simulink model "D3_LQR_1_QuadrotorModel"  (R2023b)
settings: Solver=VariableStepAuto  StartTime=0.0  StopTime=time_model  RelTol=1e-3
values from neighbouring files (symbols this model uses):
  A_flap = [c_a, c_b, 0 ... (first row only)    [LQR_calculate.m]    (also in LQR_feedback.m; LQR_linearized_test.m; MPC_test.m; MPC_test_1.m)
  A_ind = [c_d, 0, 0 ... (first row only)    [LQR_calculate.m]    (also in LQR_feedback.m; LQR_linearized_test.m; MPC_test.m; MPC_test_1.m)
  C_drag = 0    [LQR_calculate.m]    (also in LQR_feedback.m = C_drag_arr(i); LQR_linearized_test.m = C_drag_arr(i); MPC_test.m = C_drag_arr(i); MPC_test_1.m = C_drag_arr(i))
  demp = 0    [LQR_feedback.m]    (also in LQR_linearized_test.m; MPC_params.m; MPC_test_1.m; initQuadrotorData.m)
  forward_1 = 20    [LQR_feedback.m]    (also in LQR_linearized_test.m; MPC_test_1.m)
  forward_2 = 20    [LQR_feedback.m]    (also in LQR_linearized_test.m; MPC_test_1.m)
  g = 9.81    [LQR_calculate.m]    (also in LQR_feedback.m = 9.8; LQR_linearized_test.m = 9.8; LQR_testing_gpt.m; MPC_params.m = 9.8)
  Ix = m/3*a^2/12+2*0.045*l^2    (= 0.00211347222222)    [LQR_calculate.m]    (also in LQR_feedback.m; LQR_linearized_test.m; LQR_testing_gpt.m = 0.0081; MPC_params.m)
  Iy = m/3*a^2/12+4*0.045*l^2    (= 0.00413847222222)    [LQR_calculate.m]    (also in LQR_feedback.m = 0.00211347222222; LQR_linearized_test.m = 0.00211347222222; LQR_testing_gpt.m = 0.0081; MPC_params.m = 0.00211347222222)
  Iz = m/3*a^2/4+2*0.045*l^2    (= 0.00229041666667)    [LQR_calculate.m]    (also in LQR_feedback.m = 0.00431541666667; LQR_linearized_test.m = 0.00431541666667; LQR_testing_gpt.m = 0.0142; MPC_params.m = 0.00431541666667)
  J = 2.5*10^(-6)    (= 2.5e-06)    [LQR_calculate.m]    (also in LQR_feedback.m; LQR_linearized_test.m; MPC_params.m; MPC_test.m)
  K = Y * inv(P)    [LQR_calculate.m]    (also in LQR_feedback.m = [Kx;Ky;Kz;Kphi;Ktheta;-Kpsi])
  Ke = ke    (= 0.0073)    [LQR_calculate.m]    (also in LQR_feedback.m = 0.00734; LQR_linearized_test.m = 0.00734; MPC_params.m = 0.00734; MPC_test.m)
  kf = ks*r^2*airDensity*Sblade/2    (= 1.57565625e-05)    [LQR_calculate.m]    (also in LQR_feedback.m; LQR_linearized_test.m; MPC_params.m; MPC_test.m)
  Km = kt    (= 0.0073)    [LQR_calculate.m]    (also in LQR_feedback.m = 0.00734; LQR_linearized_test.m = 0.00734; MPC_params.m = 0.00734; MPC_test.m)
  kv = 1300    [LQR_feedback.m]    (also in LQR_linearized_test.m; MPC_test_1.m; initQuadrotorData.m)
  L = La    (= 5e-05)    [LQR_calculate.m]    (also in LQR_feedback.m = 0.0001; LQR_linearized_test.m = 0.0001; MPC_params.m = 0.0001; MPC_test.m)
  l = 0.15    [LQR_calculate.m]    (also in LQR_feedback.m; LQR_linearized_test.m; MPC_params.m; MPC_test.m)
  m = size(B, 2)    [LQR_calculate.m]    (also in LQR_feedback.m = 0.65; LQR_linearized_test.m = 0.65; LQR_testing_gpt.m = 1; MPC_params.m = 0.65)
  Mode = 3    [LQR_feedback.m]    (also in LQR_linearized_test.m; MPC_test_1.m = 1)
  phi0 = 0    [LQR_feedback.m]    (also in LQR_linearized_test.m; MPC_test_1.m)
  psi0 = pi/2    (= 1.57079632679)    [LQR_feedback.m]    (also in LQR_linearized_test.m; MPC_test_1.m = 0)
  R = eye(4)    [LQR_calculate.m]    (also in LQR_feedback.m = 0.058; LQR_linearized_test.m = 0.058; LQR_testing_gpt.m = diag([0.1, 10, 100, 10]); MPC_params.m = 0.058)
  rho = 1.225    [LQR_calculate.m]    (also in LQR_feedback.m; LQR_linearized_test.m; MPC_params.m; MPC_test.m)
  S = l*c*4+a*b    (= 0.0169)    [LQR_calculate.m]    (also in LQR_feedback.m; LQR_linearized_test.m; MPC_params.m; MPC_test.m)
  theta0 = 0    [LQR_feedback.m]    (also in LQR_linearized_test.m; MPC_test_1.m)
  total_time = 60    [LQR_feedback.m]    (also in LQR_linearized_test.m; MPC_test_1.m)
  up_down = 5    [LQR_feedback.m]    (also in LQR_linearized_test.m; MPC_test_1.m)
  x0 = 0    [LQR_feedback.m]    (also in LQR_linearized_test.m; MPC_test_1.m; init_nmpc.m = zeros(nx,1))
  y0 = 0    [LQR_feedback.m]    (also in LQR_linearized_test.m; MPC_test_1.m)
  z0 = 0    [LQR_feedback.m]    (also in LQR_linearized_test.m; MPC_test_1.m)
libraries: vrlib x2, sharedtransform x1
settings Model: Creator=Degra  LastModifiedBy=Degra

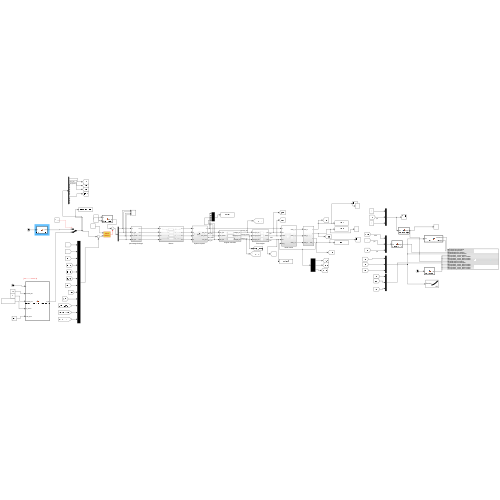
[thumbnail: Simulink's stored preview of the top-level diagram]
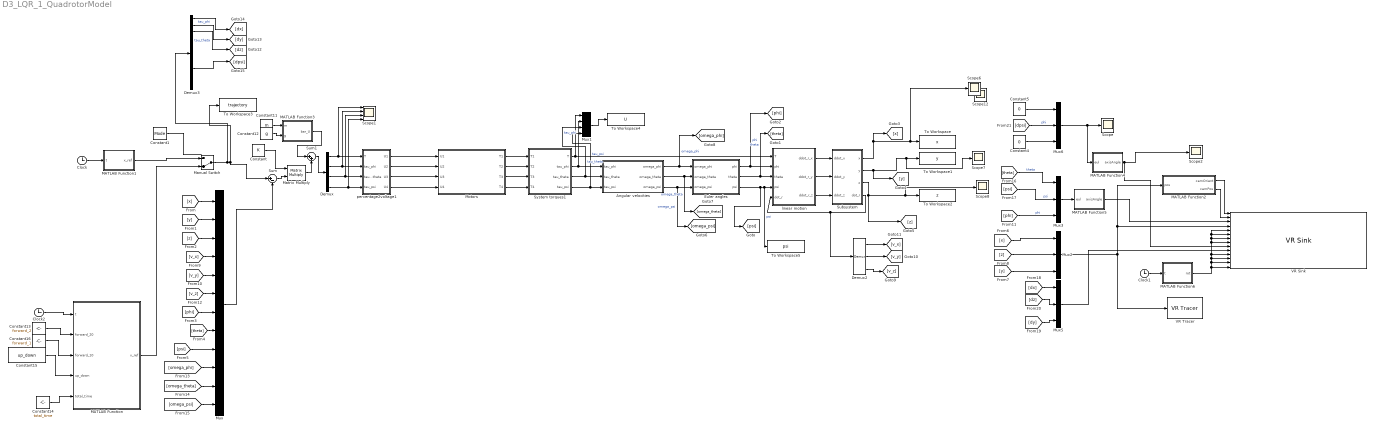
== system D3_LQR_1_QuadrotorModel ==
  Angular velocities : Subsystem
  Clock : Clock
  Clock1 : Clock
  Clock2 : Clock
  Constant : Constant  Value=K
  Constant1 : Constant  Value=Mode
  Constant11 : Constant  Value=m
  Constant12 : Constant  Value=g
  Constant13 : Constant  Value=forward_2
  Constant14 : Constant  Value=total_time
  Constant15 : Constant  Value=up_down
  Constant16 : Constant  Value=forward_1
  Constant4 : Constant  Value=0
  Constant5 : Constant  Value=0
  Demux : Demux
  Demux2 : Demux  Outputs=3
  Demux3 : Demux  Outputs=12
  Euler angles : Subsystem
  MATLAB Function : MATLAB Function  TreatAsAtomicUnit=on
  MATLAB Function1 : MATLAB Function  TreatAsAtomicUnit=on
  MATLAB Function2 : MATLAB Function  TreatAsAtomicUnit=on
  MATLAB Function3 : MATLAB Function  TreatAsAtomicUnit=on
  MATLAB Function4 : MATLAB Function  TreatAsAtomicUnit=on
  MATLAB Function5 : MATLAB Function  TreatAsAtomicUnit=on
  MATLAB Function6 : MATLAB Function  TreatAsAtomicUnit=on
  Manual Switch : ManualSwitch  CurrentSetting=0
  Matrix Multiply : Product  Multiplication=Matrix(*)
  Motors : Subsystem
  Mux : Mux  Inputs=12
  Mux1 : Mux
  Mux{2..3,5..6} (4 alike) : Mux  Inputs=3
  Scope{,2,6..8,12} (6 alike) : Scope
  Scope1 : Scope  NumInputPorts=4
  Subsystem : Subsystem
  Sum : Sum  Inputs=|+-
  Sum1 : Sum  Inputs=|++
  System torques1 : Subsystem
  To Workspace : ToWorkspace  VariableName=x  SaveFormat=Timeseries  SampleTime=-1
  To Workspace1 : ToWorkspace  VariableName=y  SaveFormat=Timeseries  SampleTime=-1
  To Workspace2 : ToWorkspace  VariableName=z  SaveFormat=Timeseries  SampleTime=-1
  To Workspace3 : ToWorkspace  VariableName=trajectory  SaveFormat=Timeseries  SampleTime=-1
  To Workspace4 : ToWorkspace  VariableName=U  SaveFormat=Timeseries  SampleTime=-1
  To Workspace5 : ToWorkspace  VariableName=psi  SaveFormat=Timeseries  SampleTime=-1
  VR Sink : vrlib/VR Sink  InstantiateOnLoad=on  SampleTime=0.1  ViewEnable=on  RemoteChange=off  RemoteView=off  FieldsWritten=FollowCam.orientation.4.1.1.double#FollowCam.position.3.1.1.double#RealQuadrotor.rotation.4.1.1.double#RealQuadrotor.translation.3.1.1.double#Propeller5_center.rotation.4.1.1.double#Propeller5_center_0001.rotation.4.1.1.double#Propeller5_center_0002.rotation.4.1.1.double#Propeller5_center_0003.rotation.4.1.1.double#IdelQuadrotor.rotation.4.1.1.double#IdelQuadrotor.translation.3.1.1.double#Propeller5_center_0004.rotation.4.1.1.double#Propeller5_center_0005.rotation.4.1.1.double#Propeller5_center_0006.rotation.4.1.1.double#Propeller5_center_0007.rotation.4.1.1.double  WorldFileName=quardrotor_space_2.x3d  WorldDescription=Aerodrome in the Desert  AutoView=off  VideoDimensions=[]  AllowVariableSize=off  FigureProperties="{'Position', 'Name', 'Viewpoint', 'CameraBound', 'CameraDirection', 'CameraPosition', 'CameraUpVector', 'ZoomFactor', 'Antialiasing', 'Headlight', 'Lighting', 'NavPanel', 'Sound', 'StatusBar', 'Stereo3D', 'Stereo3DCameraOffset', 'Stereo3DHIT', 'ToolBar', 'Textures', 'Transparency', 'Triad', 'Wireframe', 'NavZones', 'NavMode', 'NavSpeed', 'CaptureFileFormat', 'CaptureFileName', 'Record2DCompressMethod', 'Record2DCompressQuality', 'Record2D', 'Record2DFileName', 'Record2DFPS'; [1.0000000000000000e+00   7.6000000000000000e+01   1.9200000000000000e+03   9.1300000000000000e+02], 'Aerodrome in the Desert', '_untitled_3', 'on', [0.0000000000000000e+00   0.0000000000000000e+00  -1.0000000000000000e+00], [0.0000000000000000e+00   0.0000000000000000e+00   0.0000000000000000e+00], [0.0000000000000000e+00   1.0000000000000000e+00   0.0000000000000000e+00], [1.0000000000000000e+00], 'on', 'on', 'on', 'halfbar', 'on', 'on', 'off', [1.0000000149011612e-01], [0.0000000000000000e+00], 'on', 'on', 'on', 'none', 'off', 'off', 'fly', 'normal', 'tif', '%f_anim_%n.tif', 'auto', [7.5000000000000000e+01], 'on', '%f_anim_%n.avi', 'auto'}"
  VR Tracer : vrlib/VR Tracer  VrmlFile=quardrotor_space_2.x3d  MarkerName=Sphere  UseLines=on  UseTriads=on  MarkerScale=[0.01 0.01 0.01]  MarkerColorSelection=Defined as RGB values  MarkerColor=red  rgbval=[1 0 0]  Ts=0.5  ForceViewerOpen=off  ConnectPlane=off  PlaneCoeff=[0 1 0 0]  ConnectPoint=None  PointCoord=[0 0 0]
  linear motion : Subsystem
  percentage2voltage1 : Subsystem
  wires:
  Angular velocities/1(omega_phi) -> [omega_phi], Euler angles/1(omega_phi)  "omega_phi"
  Angular velocities/2(omega_theta) -> [omega_theta], Euler angles/2(omega_theta)  "omega_theta"
  Angular velocities/3(omega_psi) -> [omega_psi], Euler angles/3(omega_psi)  "omega_psi"
  Euler angles/1(phi) -> [phi], linear motion/2(phi)  "phi"
  Euler angles/2(theta) -> [theta], linear motion/3(theta)  "theta"
  Euler angles/3(psi) -> [psi], To Workspace5/1, linear motion/4(psi)  "psi"
  linear motion/1(ddot_r_x) -> Subsystem/1(ddot_x)
  linear motion/2(ddot_r_y) -> Subsystem/2(ddot_y)
  linear motion/3(ddot_r_z) -> Subsystem/3(ddot_z)
  Subsystem/1(x) -> [x], Scope6/1, To Workspace/1
  Subsystem/2(y) -> [y], Scope7/1, To Workspace1/1
  Subsystem/3(z) -> [z], Scope8/1, To Workspace2/1
  Clock/1 -> MATLAB Function1/1(t)
  [x] -> Mux/1
  [z] -> Mux/3
  [y] -> Mux/2
  Mux/1 -> Sum/2
  [phi] -> Mux/7
  [theta] -> Mux/8
  [psi] -> Mux/9
  [omega_theta] -> Mux/11
  [omega_phi] -> Mux/10
  [omega_psi] -> Mux/12
  [v_z] -> Mux/6
  [v_y] -> Mux/5
  [v_x] -> Mux/4
  Constant/1 -> Matrix Multiply/1
  Sum/1 -> Matrix Multiply/2
  MATLAB Function1/1(x_ref) -> Manual Switch/1
  Constant1/1 -> ?
  ? -> ?
  Demux/1 -> percentage2voltage1/1(T), Scope1/1
  Demux/2 -> percentage2voltage1/2(tau_phi), Scope1/2
  Demux/3 -> percentage2voltage1/3(tau_theta), Scope1/3
  Demux/4 -> percentage2voltage1/4(tau_psi), Scope1/4
  Matrix Multiply/1 -> Sum1/2
  Constant11/1 -> MATLAB Function3/1(m)
  Constant12/1 -> MATLAB Function3/2(g)
  Sum1/1 -> Demux/1
  MATLAB Function3/1(bar_U) -> Sum1/1
  MATLAB Function/1(x_ref) -> Manual Switch/2
  Constant13/1 -> MATLAB Function/2(forward_20)
  Constant16/1 -> MATLAB Function/3(forward_10)
  Constant15/1 -> MATLAB Function/4(up_down)
  Constant14/1 -> MATLAB Function/5(total_time)
  Clock2/1 -> MATLAB Function/1(t)
  Subsystem/4(dot_r) -> Demux2/1, linear motion/5(dot_r)
  Demux2/3 -> [v_z]
  Demux2/2 -> [v_y]
  Demux2/1 -> [v_x]
  System torques1/4(tau_psi) -> Mux1/4, Angular velocities/3(tau_psi)  "tau_psi"
  System torques1/3(tau_theta) -> Mux1/3, Angular velocities/2(tau_theta)  "tau_theta"
  System torques1/2(tau_phi) -> Mux1/2, Angular velocities/1(tau_phi)  "tau_phi"
  System torques1/1(T) -> Mux1/1, linear motion/1(T)
  Motors/1(T1) -> System torques1/1(T1)
  Motors/2(T2) -> System torques1/2(T2)
  Motors/3(T3) -> System torques1/3(T3)
  Motors/4(T4) -> System torques1/4(T4)
  percentage2voltage1/1(U1) -> Motors/1(U1)
  percentage2voltage1/2(U2) -> Motors/2(U2)
  percentage2voltage1/3(U3) -> Motors/3(U3)
  percentage2voltage1/4(U4) -> Motors/4(U4)
  Mux1/1 -> To Workspace4/1
  [x] -> Mux2/1
  [y] -> Mux2/3
  [z] -> Mux2/2
  [phi] -> Mux3/3  "phi"
  Manual Switch/1 -> Demux3/1, Sum/1, To Workspace3/1
  Demux3/3 -> [dz]  "tau_theta"
  Demux3/2 -> [dy]  "tau_phi"
  Demux3/1 -> [dx]
  [dz] -> Mux5/2
  [dy] -> Mux5/3
  [dx] -> Mux5/1
  Mux6/1 -> MATLAB Function4/1(eul), Scope/1
  Mux3/1 -> MATLAB Function5/1(eul)
  Demux3/9 -> [dpsi]
  Constant5/1 -> Mux6/1
  Constant4/1 -> Mux6/3
  MATLAB Function4/1(axisAngle) -> VR Sink/9, Scope2/1
  [psi] -> Mux3/2  "psi"
  [theta] -> Mux3/1  "theta"
  Clock1/1 -> MATLAB Function6/1(t)
  Mux5/1 -> VR Sink/10
  MATLAB Function2/1(camOrient) -> VR Sink/1
  MATLAB Function2/2(camPos) -> VR Sink/2
  MATLAB Function5/1(axisAngle) -> VR Sink/3
  Mux2/1 -> VR Tracer/1, VR Sink/4, MATLAB Function2/1(pos)
  MATLAB Function6/1(rot) -> VR Sink/12, VR Sink/11, VR Sink/8, VR Sink/7, VR Sink/5, VR Sink/6, VR Sink/13, VR Sink/14
  [dpsi] -> Mux6/2  "phi"

== system D3_LQR_1_QuadrotorModel/Angular velocities ==
  tau_phi : Inport
  tau_theta : Inport  Port=2
  tau_psi : Inport  Port=3
  Subsystem1 : Subsystem
  Subsystem2 : Subsystem
  Subsystem3 : Subsystem
  omega_phi : Outport
  omega_theta : Outport  Port=2
  omega_psi : Outport  Port=3
  wires:
  Subsystem2/1(omega_theta) -> omega_theta/1, Subsystem1/2(omega_theta), Subsystem3/3(omega_theta)  "omega_theta"
  tau_theta/1 -> Subsystem2/1(tau_theta)
  Subsystem1/1(omega_phi) -> omega_phi/1, Subsystem3/2(omega_phi), Subsystem2/2(omega_phi)  "omega_phi"
  Subsystem3/1(omega_psi) -> omega_psi/1, Subsystem2/3(omega_psi), Subsystem1/3(omega_psi)  "omega_psi"
  tau_phi/1 -> Subsystem1/1(tau_phi)
  tau_psi/1 -> Subsystem3/1(tau_psi)

== system D3_LQR_1_QuadrotorModel/Euler angles ==
  omega_phi : Inport
  omega_theta : Inport  Port=2
  omega_psi : Inport  Port=3
  Subsystem1 : Subsystem
  Subsystem2 : Subsystem
  Subsystem3 : Subsystem
  phi : Outport
  theta : Outport  Port=2
  psi : Outport  Port=3
  wires:
  Subsystem2/1(theta) -> theta/1, Subsystem1/2(theta), Subsystem3/4(theta)  "theta"
  Subsystem1/1(phi) -> phi/1, Subsystem3/1(phi), Subsystem2/1(phi)  "phi"
  omega_theta/1 -> Subsystem3/2(omega_theta), Subsystem1/3(omega_theta), Subsystem2/2(omega_theta)
  omega_psi/1 -> Subsystem2/3(omega_psi), Subsystem3/3(omega_psi), Subsystem1/4(omega_psi)
  omega_phi/1 -> Subsystem1/1(omega_phi)
  Subsystem3/1(psi) -> psi/1  "psi"

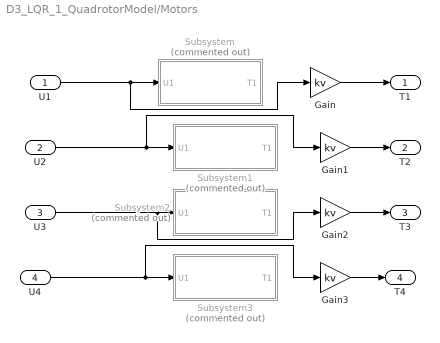
== system D3_LQR_1_QuadrotorModel/Motors ==
  U1 : Inport
  U2 : Inport  Port=2
  U3 : Inport  Port=3
  U4 : Inport  Port=4
  Gain{,1..3} (4 alike) : Gain  Gain=kv
  Subsystem : Subsystem  Commented=on
  Subsystem1 : Subsystem  Commented=on
  Subsystem2 : Subsystem  Commented=on
  Subsystem3 : Subsystem  Commented=on
  T1 : Outport
  T2 : Outport  Port=2
  T3 : Outport  Port=3
  T4 : Outport  Port=4
  wires:
  U4/1 -> Gain3/1, Subsystem3/1(U1)
  U1/1 -> Gain/1, Subsystem/1(U1)
  U3/1 -> Gain2/1, Subsystem2/1(U1)
  U2/1 -> Gain1/1, Subsystem1/1(U1)
  Gain/1 -> T1/1
  Gain1/1 -> T2/1
  Gain2/1 -> T3/1
  Gain3/1 -> T4/1

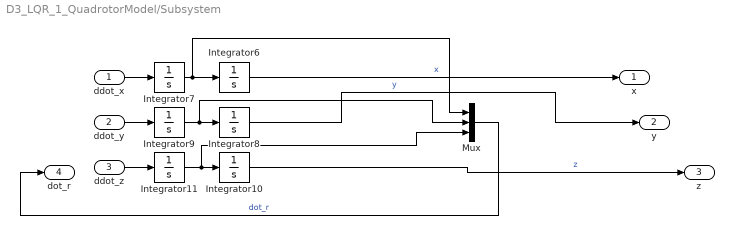
== system D3_LQR_1_QuadrotorModel/Subsystem ==
  ddot_x : Inport
  ddot_y : Inport  Port=2
  ddot_z : Inport  Port=3
  Integrator10 : Integrator  InitialCondition=z0
  Integrator11 : Integrator
  Integrator6 : Integrator  InitialCondition=x0
  Integrator7 : Integrator
  Integrator8 : Integrator  InitialCondition=y0
  Integrator9 : Integrator
  Mux : Mux  Inputs=3
  x : Outport
  y : Outport  Port=2
  z : Outport  Port=3
  dot_r : Outport  Port=4
  wires:
  Integrator9/1 -> Mux/2, Integrator8/1
  Integrator7/1 -> Mux/1, Integrator6/1
  Integrator10/1 -> z/1  "z"
  Integrator11/1 -> Mux/3, Integrator10/1
  Integrator8/1 -> y/1  "y"
  ddot_x/1 -> Integrator7/1
  Mux/1 -> dot_r/1  "dot_r"
  Integrator6/1 -> x/1  "x"
  ddot_y/1 -> Integrator9/1
  ddot_z/1 -> Integrator11/1

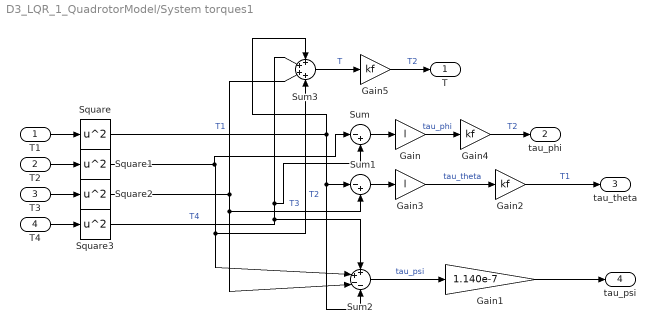
== system D3_LQR_1_QuadrotorModel/System torques1 ==
  T1 : Inport
  T2 : Inport  Port=2
  T3 : Inport  Port=3
  T4 : Inport  Port=4
  Gain : Gain  Gain=l
  Gain1 : Gain  Gain=1.140e-7
  Gain2 : Gain  Gain=kf
  Gain3 : Gain  Gain=l
  Gain4 : Gain  Gain=kf
  Gain5 : Gain  Gain=kf
  Square{,1..3} (4 alike) : Math  Operator=square
  Sum : Sum  Inputs=|-+
  Sum1 : Sum  Inputs=|-+
  Sum2 : Sum  Inputs=++--
  Sum3 : Sum  Inputs=++++
  T : Outport
  tau_phi : Outport  Port=2
  tau_theta : Outport  Port=3
  tau_psi : Outport  Port=4
  wires:
  T3/1 -> Square2/1
  T4/1 -> Square3/1
  Sum2/1 -> Gain1/1  "tau_psi"
  T1/1 -> Square/1
  Sum/1 -> Gain/1
  Sum1/1 -> Gain3/1
  Sum3/1 -> Gain5/1  "T"
  T2/1 -> Square1/1
  Gain3/1 -> Gain2/1  "tau_theta"
  Gain/1 -> Gain4/1  "tau_phi"
  Gain1/1 -> tau_psi/1
  Square/1 -> Sum1/1, Sum2/4, Sum3/1  "T1"
  Square1/1 -> Sum/1, Sum2/2, Sum3/4  "T2"
  Square2/1 -> Sum1/2, Sum2/3, Sum3/3  "T3"
  Square3/1 -> Sum/2, Sum3/2, Sum2/1  "T4"
  Gain4/1 -> tau_phi/1  "T2"
  Gain2/1 -> tau_theta/1  "T1"
  Gain5/1 -> T/1  "T2"

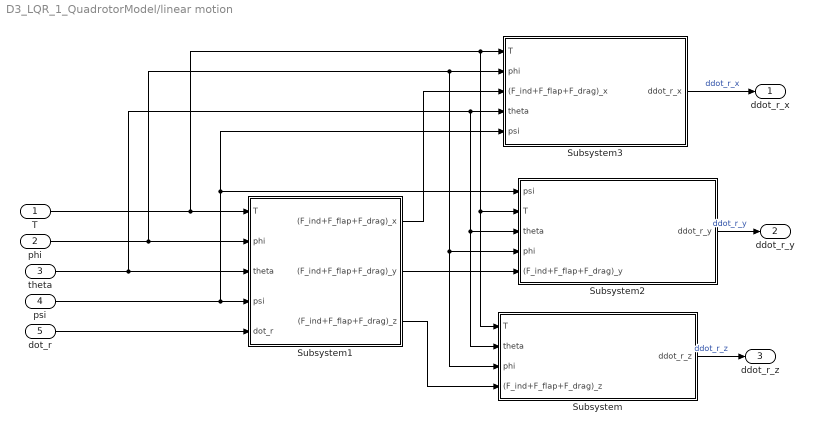
== system D3_LQR_1_QuadrotorModel/linear motion ==
  T : Inport
  phi : Inport  Port=2
  theta : Inport  Port=3
  psi : Inport  Port=4
  dot_r : Inport  Port=5
  Subsystem : Subsystem
  Subsystem1 : Subsystem
  Subsystem2 : Subsystem
  Subsystem3 : Subsystem
  ddot_r_x : Outport
  ddot_r_y : Outport  Port=2
  ddot_r_z : Outport  Port=3
  wires:
  T/1 -> Subsystem/1(T), Subsystem2/2(T), Subsystem3/1(T), Subsystem1/1(T)
  theta/1 -> Subsystem/2(theta), Subsystem2/3(theta), Subsystem3/4(theta), Subsystem1/3(theta)
  phi/1 -> Subsystem/3(phi), Subsystem2/4(phi), Subsystem3/2(phi), Subsystem1/2(phi)
  Subsystem1/3((F_ind+F_flap+F_drag)_z) -> Subsystem/4((F_ind+F_flap+F_drag)_z)
  psi/1 -> Subsystem3/5(psi), Subsystem2/1(psi), Subsystem1/4(psi)
  dot_r/1 -> Subsystem1/5(dot_r)
  Subsystem1/2((F_ind+F_flap+F_drag)_y) -> Subsystem2/5((F_ind+F_flap+F_drag)_y)
  Subsystem1/1((F_ind+F_flap+F_drag)_x) -> Subsystem3/3((F_ind+F_flap+F_drag)_x)
  Subsystem3/1(ddot_r_x) -> ddot_r_x/1  "ddot_r_x"
  Subsystem2/1(ddot_r_y) -> ddot_r_y/1  "ddot_r_y"
  Subsystem/1(ddot_r_z) -> ddot_r_z/1  "ddot_r_z"

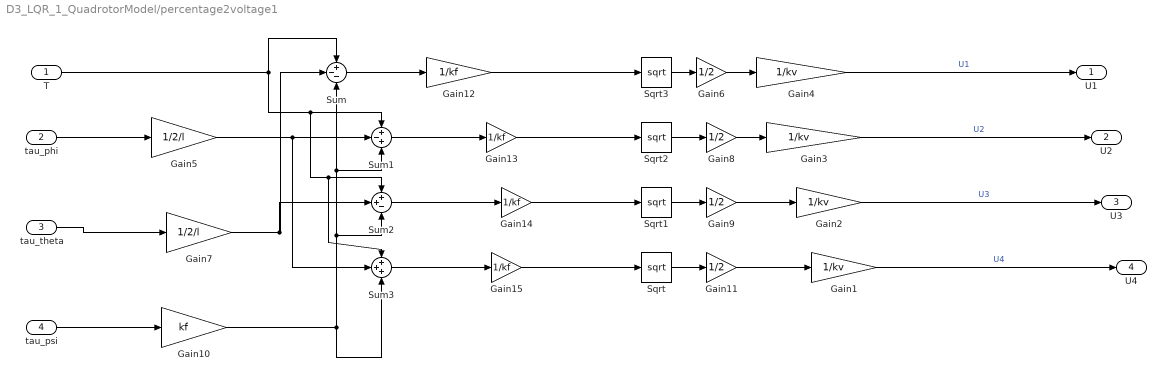
== system D3_LQR_1_QuadrotorModel/percentage2voltage1 ==
  T : Inport
  tau_phi : Inport  Port=2
  tau_theta : Inport  Port=3
  tau_psi : Inport  Port=4
  Gain{1..4} (4 alike) : Gain  Gain=1/kv
  Gain10 : Gain  Gain=kf
  Gain{6,8..9,11} (4 alike) : Gain  Gain=1/2
  Gain{12..15} (4 alike) : Gain  Gain=1/kf
  Gain5 : Gain  Gain=1/2/l
  Gain7 : Gain  Gain=1/2/l
  Sqrt{,1..3} (4 alike) : Sqrt
  Sum : Sum  Inputs=+--
  Sum1 : Sum  Inputs=+-+
  Sum2 : Sum  Inputs=++-
  Sum3 : Sum  Inputs=+++
  U1 : Outport
  U2 : Outport  Port=2
  U3 : Outport  Port=3
  U4 : Outport  Port=4
  wires:
  Gain2/1 -> U3/1  "U3"
  Gain4/1 -> U1/1  "U1"
  Gain3/1 -> U2/1  "U2"
  Gain1/1 -> U4/1  "U4"
  Sum3/1 -> Gain15/1
  Sum2/1 -> Gain14/1
  tau_phi/1 -> Gain5/1
  tau_theta/1 -> Gain7/1
  tau_psi/1 -> Gain10/1
  Gain10/1 -> Sum3/3, Sum1/3, Sum/3, Sum2/3
  Sqrt/1 -> Gain11/1
  Sqrt1/1 -> Gain9/1
  Sqrt2/1 -> Gain8/1
  Sqrt3/1 -> Gain6/1
  Gain6/1 -> Gain4/1
  Gain8/1 -> Gain3/1
  Gain9/1 -> Gain2/1
  Gain11/1 -> Gain1/1
  Sum/1 -> Gain12/1
  Sum1/1 -> Gain13/1
  Gain14/1 -> Sqrt1/1
  Gain15/1 -> Sqrt/1
  Gain5/1 -> Sum3/2, Sum1/2
  Gain7/1 -> Sum2/2, Sum/2
  T/1 -> Sum3/1, Sum2/1, Sum1/1, Sum/1
  Gain12/1 -> Sqrt3/1
  Gain13/1 -> Sqrt2/1

== system D3_LQR_1_QuadrotorModel/Angular velocities/Subsystem1 ==
  tau_phi : Inport
  omega_theta : Inport  Port=2
  omega_psi : Inport  Port=3
  Gain : Gain  Gain=Iy-Iz
  Gain1 : Gain  Gain=1/Ix
  Integrator12 : Integrator
  Product : Product
  Sum : Sum  Inputs=|++
  omega_phi : Outport
  wires:
  Gain/1 -> Sum/2
  omega_theta/1 -> Product/1
  Product/1 -> Gain/1
  Sum/1 -> Gain1/1  "dot_omega_phi"
  tau_phi/1 -> Sum/1
  omega_psi/1 -> Product/2
  Gain1/1 -> Integrator12/1
  Integrator12/1 -> omega_phi/1  "omega_phi"

== system D3_LQR_1_QuadrotorModel/Angular velocities/Subsystem2 ==
  tau_theta : Inport
  omega_phi : Inport  Port=2
  omega_psi : Inport  Port=3
  Gain : Gain  Gain=Iz-Ix
  Gain1 : Gain  Gain=1/Iy
  Integrator12 : Integrator
  Product : Product
  Sum : Sum  Inputs=|++
  omega_theta : Outport
  wires:
  Gain/1 -> Sum/2
  Sum/1 -> Gain1/1  "omega_theta"
  omega_phi/1 -> Product/1
  Product/1 -> Gain/1
  tau_theta/1 -> Sum/1
  omega_psi/1 -> Product/2
  Gain1/1 -> Integrator12/1
  Integrator12/1 -> omega_theta/1  "omega_theta"

== system D3_LQR_1_QuadrotorModel/Angular velocities/Subsystem3 ==
  tau_psi : Inport
  omega_phi : Inport  Port=2
  omega_theta : Inport  Port=3
  Gain : Gain  Gain=Ix-Iy
  Gain1 : Gain  Gain=1/Iz
  Integrator12 : Integrator
  Product : Product
  Sum : Sum  Inputs=|++
  omega_psi : Outport
  wires:
  Gain/1 -> Sum/2
  omega_phi/1 -> Product/1
  Product/1 -> Gain/1
  Sum/1 -> Gain1/1  "dot_omega_psi"
  tau_psi/1 -> Sum/1
  omega_theta/1 -> Product/2
  Gain1/1 -> Integrator12/1
  Integrator12/1 -> omega_psi/1  "omega_psi"

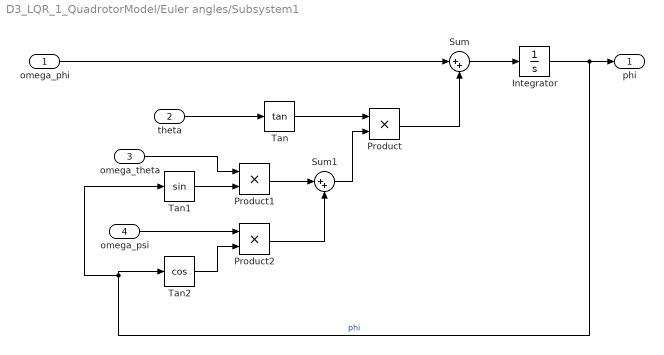
== system D3_LQR_1_QuadrotorModel/Euler angles/Subsystem1 ==
  omega_phi : Inport
  theta : Inport  Port=2
  omega_theta : Inport  Port=3
  omega_psi : Inport  Port=4
  Integrator : Integrator  InitialCondition=phi0
  Product : Product
  Product1 : Product
  Product2 : Product
  Sum : Sum  Inputs=|++
  Sum1 : Sum  Inputs=|++
  Tan : Trigonometry  Operator=tan
  Tan1 : Trigonometry
  Tan2 : Trigonometry  Operator=cos
  phi : Outport
  wires:
  Product2/1 -> Sum1/2
  Tan1/1 -> Product1/2
  Sum/1 -> Integrator/1
  Sum1/1 -> Product/2
  Tan/1 -> Product/1
  Tan2/1 -> Product2/2
  Product1/1 -> Sum1/1
  omega_psi/1 -> Product2/1
  omega_theta/1 -> Product1/1
  Integrator/1 -> Tan1/1, Tan2/1, phi/1  "phi"
  theta/1 -> Tan/1
  omega_phi/1 -> Sum/1
  Product/1 -> Sum/2

== system D3_LQR_1_QuadrotorModel/Euler angles/Subsystem2 ==
  phi : Inport
  omega_theta : Inport  Port=2
  omega_psi : Inport  Port=3
  Integrator : Integrator  InitialCondition=theta0
  Product1 : Product
  Product2 : Product
  Sum1 : Sum  Inputs=|+-
  Tan1 : Trigonometry  Operator=cos
  Tan2 : Trigonometry
  theta : Outport
  wires:
  Product2/1 -> Sum1/2
  Tan1/1 -> Product1/2
  Tan2/1 -> Product2/2
  Product1/1 -> Sum1/1
  omega_psi/1 -> Product2/1
  Integrator/1 -> theta/1  "theta"
  phi/1 -> Tan2/1, Tan1/1
  omega_theta/1 -> Product1/1
  Sum1/1 -> Integrator/1

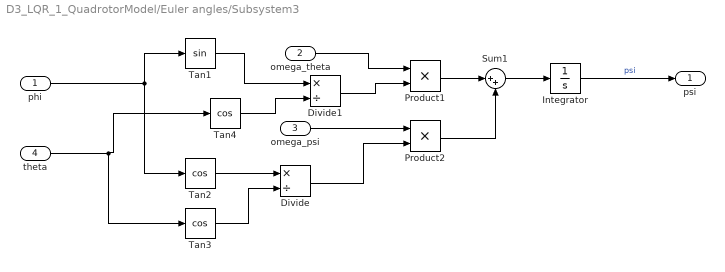
== system D3_LQR_1_QuadrotorModel/Euler angles/Subsystem3 ==
  phi : Inport
  omega_theta : Inport  Port=2
  omega_psi : Inport  Port=3
  theta : Inport  Port=4
  Divide : Product  Inputs=*/
  Divide1 : Product  Inputs=*/
  Integrator : Integrator  InitialCondition=psi0
  Product1 : Product
  Product2 : Product
  Sum1 : Sum  Inputs=|++
  Tan1 : Trigonometry
  Tan2 : Trigonometry  Operator=cos
  Tan3 : Trigonometry  Operator=cos
  Tan4 : Trigonometry  Operator=cos
  psi : Outport
  wires:
  Product2/1 -> Sum1/2
  Product1/1 -> Sum1/1
  omega_psi/1 -> Product2/1
  Integrator/1 -> psi/1  "psi"
  phi/1 -> Tan1/1, Tan2/1
  theta/1 -> Tan4/1, Tan3/1
  Divide/1 -> Product2/2
  Tan2/1 -> Divide/1
  Tan3/1 -> Divide/2
  Divide1/1 -> Product1/2
  Tan1/1 -> Divide1/1
  Tan4/1 -> Divide1/2
  omega_theta/1 -> Product1/1
  Sum1/1 -> Integrator/1

== system D3_LQR_1_QuadrotorModel/Motors/Subsystem ==
  U1 : Inport
  Add : Sum  Inputs=+--
  Add1 : Sum  Inputs=+-
  Gain : Gain  Gain=demp
  Gain1 : Gain  Gain=Km
  Gain2 : Gain  Gain=1/L
  Gain3 : Gain  Gain=Ke
  Gain5 : Gain  Gain=R
  Gain6 : Gain  Gain=1/J
  Integrator : Integrator
  Integrator1 : Integrator
  T1 : Outport
  wires:
  Gain2/1 -> Integrator/1
  Add/1 -> Gain2/1
  Integrator/1 -> Gain1/1, Gain5/1
  Gain5/1 -> Add/3
  U1/1 -> Add/1
  Gain1/1 -> Add1/1
  Add1/1 -> Gain6/1
  Integrator1/1 -> T1/1, Gain3/1, Gain/1
  Gain3/1 -> Add/2
  Gain/1 -> Add1/2
  Gain6/1 -> Integrator1/1

== system D3_LQR_1_QuadrotorModel/Motors/Subsystem1 ==
  U1 : Inport
  Add : Sum  Inputs=+--
  Add1 : Sum  Inputs=+-
  Gain : Gain  Gain=demp
  Gain1 : Gain  Gain=Km
  Gain2 : Gain  Gain=1/L
  Gain3 : Gain  Gain=Ke
  Gain5 : Gain  Gain=R
  Gain6 : Gain  Gain=1/J
  Integrator : Integrator
  Integrator1 : Integrator
  T1 : Outport
  wires:
  Gain2/1 -> Integrator/1
  Add/1 -> Gain2/1
  Integrator/1 -> Gain1/1, Gain5/1
  Gain5/1 -> Add/3
  U1/1 -> Add/1
  Gain1/1 -> Add1/1
  Add1/1 -> Gain6/1
  Integrator1/1 -> T1/1, Gain3/1, Gain/1
  Gain3/1 -> Add/2
  Gain/1 -> Add1/2
  Gain6/1 -> Integrator1/1

== system D3_LQR_1_QuadrotorModel/Motors/Subsystem2 ==
  U1 : Inport
  Add : Sum  Inputs=+--
  Add1 : Sum  Inputs=+-
  Gain : Gain  Gain=demp
  Gain1 : Gain  Gain=Km
  Gain2 : Gain  Gain=1/L
  Gain3 : Gain  Gain=Ke
  Gain5 : Gain  Gain=R
  Gain6 : Gain  Gain=1/J
  Integrator : Integrator
  Integrator1 : Integrator
  T1 : Outport
  wires:
  Gain2/1 -> Integrator/1
  Add/1 -> Gain2/1
  Integrator/1 -> Gain1/1, Gain5/1
  Gain5/1 -> Add/3
  U1/1 -> Add/1
  Gain1/1 -> Add1/1
  Add1/1 -> Gain6/1
  Integrator1/1 -> T1/1, Gain3/1, Gain/1
  Gain3/1 -> Add/2
  Gain/1 -> Add1/2
  Gain6/1 -> Integrator1/1

== system D3_LQR_1_QuadrotorModel/Motors/Subsystem3 ==
  U1 : Inport
  Add : Sum  Inputs=+--
  Add1 : Sum  Inputs=+-
  Gain : Gain  Gain=demp
  Gain1 : Gain  Gain=Km
  Gain2 : Gain  Gain=1/L
  Gain3 : Gain  Gain=Ke
  Gain5 : Gain  Gain=R
  Gain6 : Gain  Gain=1/J
  Integrator : Integrator
  Integrator1 : Integrator
  T1 : Outport
  wires:
  Gain2/1 -> Integrator/1
  Add/1 -> Gain2/1
  Integrator/1 -> Gain1/1, Gain5/1
  Gain5/1 -> Add/3
  U1/1 -> Add/1
  Gain1/1 -> Add1/1
  Add1/1 -> Gain6/1
  Integrator1/1 -> T1/1, Gain3/1, Gain/1
  Gain3/1 -> Add/2
  Gain/1 -> Add1/2
  Gain6/1 -> Integrator1/1

== system D3_LQR_1_QuadrotorModel/linear motion/Subsystem ==
  T : Inport
  theta : Inport  Port=2
  phi : Inport  Port=3
  (F_ind+F_flap+F_drag)_z : Inport  Port=4
  Constant4 : Constant  Value=m*g
  Cos4 : Trigonometry  Operator=cos
  Cos5 : Trigonometry  Operator=cos
  Gain4 : Gain  Gain=1/m
  Product2 : Product  Inputs=3
  Sum2 : Sum  Inputs=|+--
  ddot_r_z : Outport
  wires:
  Product2/1 -> Sum2/1
  phi/1 -> Cos4/1
  theta/1 -> Cos5/1
  T/1 -> Product2/1
  Cos4/1 -> Product2/2
  Constant4/1 -> Sum2/3
  Cos5/1 -> Product2/3
  (F_ind+F_flap+F_drag)_z/1 -> Sum2/2
  Sum2/1 -> Gain4/1
  Gain4/1 -> ddot_r_z/1  "ddot_r_z"

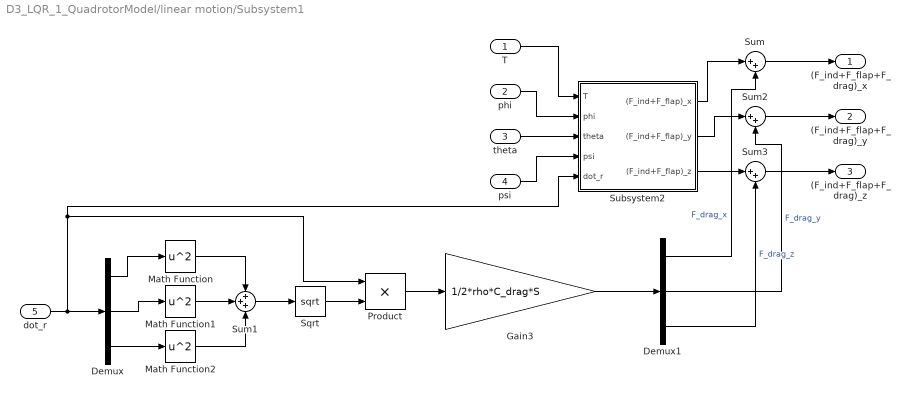
== system D3_LQR_1_QuadrotorModel/linear motion/Subsystem1 ==
  T : Inport
  phi : Inport  Port=2
  theta : Inport  Port=3
  psi : Inport  Port=4
  dot_r : Inport  Port=5
  Demux : Demux  Outputs=3
  Demux1 : Demux  Outputs=3
  Gain3 : Gain  Gain=1/2*rho*C_drag*S
  Math Function : Math  Operator=square
  Math Function1 : Math  Operator=square
  Math Function2 : Math  Operator=square
  Product : Product
  Sqrt : Sqrt
  Subsystem2 : Subsystem
  Sum : Sum  Inputs=|++
  Sum1 : Sum  Inputs=+++
  Sum2 : Sum  Inputs=|++
  Sum3 : Sum  Inputs=|++
  (F_ind+F_flap+F_drag)_x : Outport
  (F_ind+F_flap+F_drag)_y : Outport  Port=2
  (F_ind+F_flap+F_drag)_z : Outport  Port=3
  wires:
  Demux1/2 -> Sum2/2  "F_drag_y"
  dot_r/1 -> Product/1, Subsystem2/5(dot_r), Demux/1
  Math Function1/1 -> Sum1/2
  Demux/1 -> Math Function/1
  Demux/2 -> Math Function1/1
  Sum1/1 -> Sqrt/1
  Math Function/1 -> Sum1/1
  Demux/3 -> Math Function2/1
  Demux1/3 -> Sum3/2  "F_drag_z"
  Subsystem2/2((F_ind+F_flap)_y) -> Sum2/1
  Math Function2/1 -> Sum1/3
  Sqrt/1 -> Product/2
  phi/1 -> Subsystem2/2(phi)
  Product/1 -> Gain3/1
  T/1 -> Subsystem2/1(T)
  theta/1 -> Subsystem2/3(theta)
  psi/1 -> Subsystem2/4(psi)
  Gain3/1 -> Demux1/1
  Subsystem2/1((F_ind+F_flap)_x) -> Sum/1
  Subsystem2/3((F_ind+F_flap)_z) -> Sum3/1
  Demux1/1 -> Sum/2  "F_drag_x"
  Sum/1 -> (F_ind+F_flap+F_drag)_x/1
  Sum2/1 -> (F_ind+F_flap+F_drag)_y/1
  Sum3/1 -> (F_ind+F_flap+F_drag)_z/1

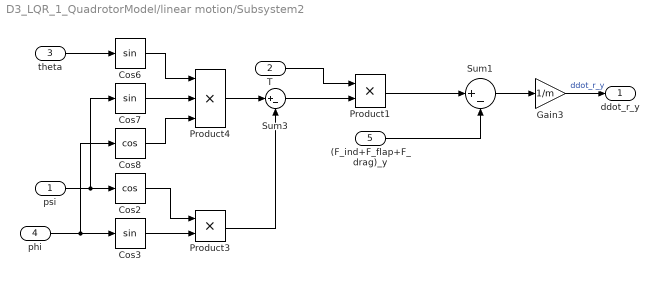
== system D3_LQR_1_QuadrotorModel/linear motion/Subsystem2 ==
  psi : Inport
  T : Inport  Port=2
  theta : Inport  Port=3
  phi : Inport  Port=4
  (F_ind+F_flap+F_drag)_y : Inport  Port=5
  Cos2 : Trigonometry  Operator=cos
  Cos3 : Trigonometry
  Cos6 : Trigonometry
  Cos7 : Trigonometry
  Cos8 : Trigonometry  Operator=cos
  Gain3 : Gain  Gain=1/m
  Product1 : Product
  Product3 : Product
  Product4 : Product  Inputs=3
  Sum1 : Sum  Inputs=|+-
  Sum3 : Sum  Inputs=|+-
  ddot_r_y : Outport
  wires:
  Cos6/1 -> Product4/1
  theta/1 -> Cos6/1
  psi/1 -> Cos7/1, Cos2/1
  Cos7/1 -> Product4/2
  Sum1/1 -> Gain3/1
  phi/1 -> Cos8/1, Cos3/1
  Cos8/1 -> Product4/3
  Cos2/1 -> Product3/1
  Cos3/1 -> Product3/2
  Product4/1 -> Sum3/1
  Product3/1 -> Sum3/2
  T/1 -> Product1/1
  Sum3/1 -> Product1/2
  Product1/1 -> Sum1/1
  (F_ind+F_flap+F_drag)_y/1 -> Sum1/2
  Gain3/1 -> ddot_r_y/1  "ddot_r_y"

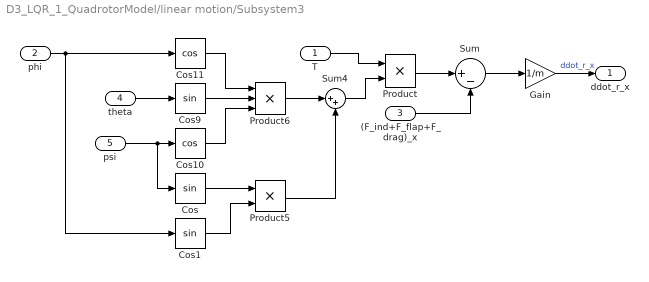
== system D3_LQR_1_QuadrotorModel/linear motion/Subsystem3 ==
  T : Inport
  phi : Inport  Port=2
  (F_ind+F_flap+F_drag)_x : Inport  Port=3
  theta : Inport  Port=4
  psi : Inport  Port=5
  Cos : Trigonometry
  Cos1 : Trigonometry
  Cos10 : Trigonometry  Operator=cos
  Cos11 : Trigonometry  Operator=cos
  Cos9 : Trigonometry
  Gain : Gain  Gain=1/m
  Product : Product
  Product5 : Product
  Product6 : Product  Inputs=3
  Sum : Sum  Inputs=|+-
  Sum4 : Sum  Inputs=|++
  ddot_r_x : Outport
  wires:
  theta/1 -> Cos9/1
  Cos/1 -> Product5/1
  psi/1 -> Cos10/1, Cos/1
  Cos11/1 -> Product6/1
  Sum/1 -> Gain/1
  (F_ind+F_flap+F_drag)_x/1 -> Sum/2
  phi/1 -> Cos11/1, Cos1/1
  Cos1/1 -> Product5/2
  Cos9/1 -> Product6/2
  Cos10/1 -> Product6/3
  Product6/1 -> Sum4/1
  Product5/1 -> Sum4/2
  T/1 -> Product/1
  Sum4/1 -> Product/2
  Product/1 -> Sum/1
  Gain/1 -> ddot_r_x/1  "ddot_r_x"

== system D3_LQR_1_QuadrotorModel/linear motion/Subsystem1/Subsystem2 ==
  T : Inport
  phi : Inport  Port=2
  theta : Inport  Port=3
  psi : Inport  Port=4
  dot_r : Inport  Port=5
  Demux : Demux  Outputs=3
  Subsystem1 : Subsystem
  (F_ind+F_flap)_x : Outport
  (F_ind+F_flap)_y : Outport  Port=2
  (F_ind+F_flap)_z : Outport  Port=3
  wires:
  T/1 -> Subsystem1/5(T)
  Subsystem1/1(F_ind+F_flap) -> Demux/1
  psi/1 -> Subsystem1/3(psi)
  Demux/2 -> (F_ind+F_flap)_y/1  "(F_ind+F_flap)_y"
  dot_r/1 -> Subsystem1/4(dot_r)
  theta/1 -> Subsystem1/2(theta)
  phi/1 -> Subsystem1/1(phi)
  Demux/1 -> (F_ind+F_flap)_x/1  "(F_ind+F_flap)_x"
  Demux/3 -> (F_ind+F_flap)_z/1  "(F_ind+F_flap)_z"

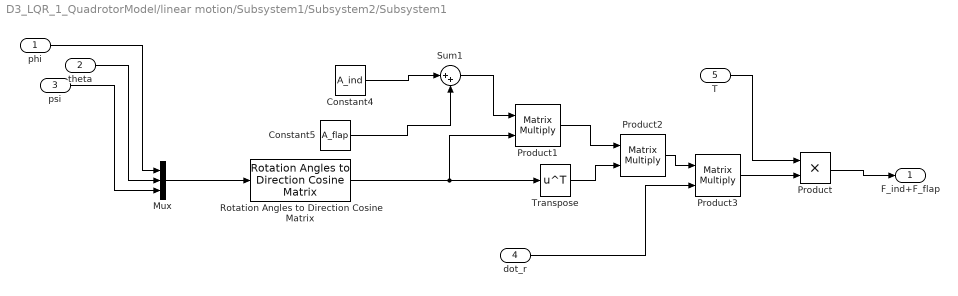
== system D3_LQR_1_QuadrotorModel/linear motion/Subsystem1/Subsystem2/Subsystem1 ==
  phi : Inport
  theta : Inport  Port=2
  psi : Inport  Port=3
  dot_r : Inport  Port=4
  T : Inport  Port=5
  Constant4 : Constant  Value=A_ind
  Constant5 : Constant  Value=A_flap
  Mux : Mux  Inputs=3
  Product : Product
  Product1 : Product  Multiplication=Matrix(*)
  Product2 : Product  Multiplication=Matrix(*)
  Product3 : Product  Multiplication=Matrix(*)
  Rotation Angles to Direction Cosine Matrix : sharedtransform/Rotation Angles to Direction Cosine Matrix  rotationOrder=ZYX  aMode=aMode
  Sum1 : Sum  Inputs=|++
  Transpose : Math  Operator=transpose
  F_ind+F_flap : Outport
  wires:
  Constant4/1 -> Sum1/1
  Product1/1 -> Product2/1
  Sum1/1 -> Product1/1
  Constant5/1 -> Sum1/2
  psi/1 -> Mux/3
  Product2/1 -> Product3/1
  Rotation Angles to Direction Cosine Matrix/1 -> Product1/2, Transpose/1
  theta/1 -> Mux/2
  Mux/1 -> Rotation Angles to Direction Cosine Matrix/1
  Transpose/1 -> Product2/2
  phi/1 -> Mux/1
  dot_r/1 -> Product3/2
  Product3/1 -> Product/2
  Product/1 -> F_ind+F_flap/1
  T/1 -> Product/1

== matlab function D3_LQR_1_QuadrotorModel/MATLAB Function1 ==
  data: t input; x_ref output size=[12 1]
function x_ref = trajectory_generator(t)
%#codegen
% Генератор траектории «восьмерка» с вычислением угла psi по направлению движения

    % Параметры восьмерки
    A = 10;      % амплитуда по x
    B = 6.5;     % амплитуда по y
    h = 5;       % постоянная высота
    w = 0.2;     % угловая частота

    % Позиция квадрокоптера
    x = A * sin(w * t);
    y = B * sin(w * t) .* cos(w * t);
    z = h;

    % Малый шаг для численного вычисления направления
    dt_small = 1e-3;
    x_next = A * sin(w * (t + dt_small));
    y_next = B * sin(w * (t + dt_small)) .* cos(w * (t + dt_small));
    
    psi = 0;
    % Направление движения (heading)
   % psi = atan2(y_next - y, x_next - x);
   % psi = wrapToPi(psi);
    % psi =    % Все скорости и угловые скорости оставляем нулевыми
    x_ref = [
        x;      % 1: x
        y;      % 2: y
        z;      % 3: z
        0;0;0;  % 4-6: vx, vy, vz
        0;0;    % 7-8: phi, theta
        psi;    % 9: psi
        0;0;0   % 10-12: w_phi, w_theta, w_psi
    ];
end

== matlab function D3_LQR_1_QuadrotorModel/MATLAB Function2 ==
  data: camOrient output; pos input; camPos output
function [camOrient,camPos] = cameraFixedLookAtAngles(pos)
% pos: [x; y; z] – позиция квадрокоптера в мировой системе
% camPos: [x; y; z] – фиксированная позиция камеры
% camOrient: [ax; ay; az; theta] – axis‑angle поворот камеры

  % === Настройки ===
  camPos = [10; 10; 10];     % ваша фикс. позиция камеры
  
  % === Вычисляем направление «взгляда» ===
  d = pos - camPos;         % вектор «квадрокоптер – камера»
  d = d / norm(d);          % нормируем

  % дефолтный вектор «вперед» в VRML (смотрит вдоль -Z)
  v0 = [0; 0; -1];          
  
  % если почти параллельны — не крутим
  if abs(dot(v0,d)) > 0.9999
    axis = [0;1;0];
    angle = 0;
  else
    % ось вращения = v0 × d
    axis = cross(v0, d);
    axis = axis / norm(axis);
    angle = acos( dot(v0, d) );
  end

  camOrient = [axis; angle];
end

== matlab function D3_LQR_1_QuadrotorModel/MATLAB Function3 ==
  data: m input; bar_U output; g input
function bar_U = trajectory_generator(m,g)
%#codegen

bar_U = [m*g; 0; 0; 0];
end

== matlab function D3_LQR_1_QuadrotorModel/MATLAB Function ==
  data: t input; forward_20 input; x_ref output size=[12 1]; forward_10 input; up_down input; total_time input
function x_ref = generate_quadcopter_route_real_time(t, forward_20, forward_10, up_down, total_time)
    % Доля времени на повороты
    turn_time_ratio = 0.2;
    total_turn_time = total_time * turn_time_ratio;
    total_linear_time = total_time - total_turn_time;

    % Время на каждый поворот
    turn_time = total_turn_time / 4;

    % Линейные сегменты разбиты на движение по XY и по Z (всего 8 отрезков)
    % Формат: [dx, dy, dz, dpsi]
    segments = [
        forward_20, 0, 0, 0;       % вперед
        0, 0, up_down, 0;          % вверх
        0, 0, 0, -pi/2;             % поворот влево
        forward_10, 0, 0, 0;       % вперед
        0, 0, -up_down, 0;         % вниз
        0, 0, 0, -pi/2;             % поворот влево
        forward_20, 0, 0, 0;       % вперед
        0, 0, up_down, 0;          % вверх
        0, 0, 0, -pi/2;             % поворот влево
        forward_10, 0, 0, 0;       % вперед
        0, 0, -up_down, 0;         % вниз
        0, 0, 0, -pi/2;             % поворот влево
    ];

    % Определяем длину каждого линейного сегмента
    segment_lengths = vecnorm(segments(:, 1:3), 2, 2);
    total_path_length = sum(segment_lengths);
    
    % Распределяем время на каждый линейный сегмент пропорционально длине
    segment_times = zeros(size(segments, 1), 1);
    for i = 1:size(segments, 1)
        if segments(i, 4) == 0 % линейное движение
            segment_times(i) = segment_lengths(i) / total_path_length * total_linear_time;
        else % поворот
            segment_times(i) = turn_time;
        end
    end

    % Инициализация
    current_x = 0;
    current_y = 0;
    current_z = 0;
    current_psi = 0;
    accumulated_time = 0;

    % Обход сегментов
    for s = 1:size(segments, 1)
        dt = segment_times(s);
        if t <= accumulated_time + dt || s == size(segments,1)
            % Текущий сегмент
            segment_progress = (t - accumulated_time) / dt;
            segment_progress = max(0, min(1, segment_progress));

            dx = segments(s, 1) * segment_progress;
            dy = segments(s, 2) * segment_progress;
            dz = segments(s, 3) * segment_progress;
            dpsi = segments(s, 4) * segment_progress;

            % Преобразование координат с учетом текущего поворота
            if dx ~= 0 || dy ~= 0
                R = [cos(current_psi), -sin(current_psi);
                     sin(current_psi),  cos(current_psi)];
                xy = R * [dx; dy];
            else
                xy = [0; 0];
            end

            x = current_x + xy(1);
            y = current_y + xy(2);
            z = current_z + dz;
            psi = current_psi + dpsi;

            x_ref = [x; y; z; 0; 0; 0; 0; 0; psi; 0; 0; 0];
            return;
        end

        % Завершённый сегмент — обновляем позицию
        dx = segments(s, 1);
        dy = segments(s, 2);
        dz = segments(s, 3);
        dpsi = segments(s, 4);

        if dx ~= 0 || dy ~= 0
            R = [cos(current_psi), -sin(current_psi);
                 sin(current_psi),  cos(current_psi)];
            xy = R * [dx; dy];
        else
            xy = [0; 0];
        end

        current_x = current_x + xy(1);
        current_y = current_y + xy(2);
        current_z = current_z + dz;
        current_psi = current_psi + dpsi;

        accumulated_time = accumulated_time + segment_times(s);
    end

    % Если всё завершено — остаёмся в конечной точке
    x_ref = [current_x; current_y; current_z; 0; 0; 0; 0; 0; current_psi; 0; 0; 0];
end

== matlab function D3_LQR_1_QuadrotorModel/MATLAB Function4 ==
  data: eul input; axisAngle output
function axisAngle = eul2AxisAngle(eul)
% eul: [phi; theta; psi] – углы Эйлера в радианах (roll, pitch, yaw)
% axisAngle: [ax; ay; az; angle] – axis‑angle, угол в рад

    % Конвертируем сначала в кватернион [w x y z]
    % MATLAB ожидает порядок [yaw pitch roll] и стандарт 'ZYX'
    q = eul2quat([eul(3), eul(2), eul(1)], 'ZYX');  
    
    % Вычисляем угол поворота
    angle = 2 * acos( q(1) );
    
    % sin(theta/2) для нормировки оси
    s = sqrt(1 - q(1)^2);
    
    if s < 1e-6
        % Угол почти нулевой — ось можно задать произвольно
        axis = [1; 0; 0];
    else
        % Нормируем вектор-проекция кватерниона
        axis = q(2:4)' / s;
    end
    
    axisAngle = [axis; angle];
end

== matlab function D3_LQR_1_QuadrotorModel/MATLAB Function5 ==
  data: eul input; axisAngle output
function axisAngle = eul2AxisAngle(eul)
% eul: [phi; theta; psi] – углы Эйлера в радианах (roll, pitch, yaw)
% axisAngle: [ax; ay; az; angle] – axis‑angle, угол в рад

    % Конвертируем сначала в кватернион [w x y z]
    % MATLAB ожидает порядок [yaw pitch roll] и стандарт 'ZYX'
    q = eul2quat([eul(3), eul(2), eul(1)], 'ZYX');  
    
    % Вычисляем угол поворота
    angle = 2 * acos( q(1) );
    
    % sin(theta/2) для нормировки оси
    s = sqrt(1 - q(1)^2);
    
    if s < 1e-6
        % Угол почти нулевой — ось можно задать произвольно
        axis = [1; 0; 0];
    else
        % Нормируем вектор-проекция кватерниона
        axis = q(2:4)' / s;
    end
    
    axisAngle = [axis; angle];
end

== matlab function D3_LQR_1_QuadrotorModel/MATLAB Function6 ==
  data: t input; rot output
function rot = rotor_angle(t)
%#codegen
    omega = 20; % рад/с
    angle = mod(omega * t, 2*pi);
    rot = [0 0 1 angle];  % вращение вокруг оси Z
end
